simulink model "qr8x8"  (R2018b)
settings: Solver=VariableStepAuto  StartTime=0.0  StopTime=10.0  RelTol=1e-3
libraries: hdlsllib x71, simulink x16, dspmathops x1
(part 2 of 2)

== system qr8x8/QRdecomp/Q_col/Subsystem5/Subsystem5 ==
  i_bit : Inport
  j_bit : Inport  Port=2
  load : Inport  Port=3
  wr_en : Inport  Port=4
  Bit Concat : hdlsllib/Logic and Bit Operations/Bit Concat  numInputs=2
      settings: SourceProductName=HDL Coder  SourceProductBaseCode=HD
  Logical Operator : Logic  Operator=OR  AllPortsSameDT=off  OutDataTypeStr=boolean
  Logical Operator1 : Logic  Operator=OR  AllPortsSameDT=off  OutDataTypeStr=boolean
  Logical Operator2 : Logic  AllPortsSameDT=off  OutDataTypeStr=boolean
  din_sel : Outport
  en : Outport  Port=2
  wires:
  i_bit/1 -> Logical Operator/1, Bit Concat/2
  Logical Operator2/1 -> en/1
  wr_en/1 -> Logical Operator2/2
  Logical Operator1/1 -> Logical Operator2/1
  load/1 -> Logical Operator1/2
  Logical Operator/1 -> Logical Operator1/1
  Bit Concat/1 -> din_sel/1
  j_bit/1 -> Bit Concat/1, Logical Operator/2

== system qr8x8/QRdecomp/Q_col/Subsystem5/Subsystem6 ==
  i_bit : Inport
  j_bit : Inport  Port=2
  load : Inport  Port=3
  wr_en : Inport  Port=4
  Bit Concat : hdlsllib/Logic and Bit Operations/Bit Concat  numInputs=2
      settings: SourceProductName=HDL Coder  SourceProductBaseCode=HD
  Logical Operator : Logic  Operator=OR  AllPortsSameDT=off  OutDataTypeStr=boolean
  Logical Operator1 : Logic  Operator=OR  AllPortsSameDT=off  OutDataTypeStr=boolean
  Logical Operator2 : Logic  AllPortsSameDT=off  OutDataTypeStr=boolean
  din_sel : Outport
  en : Outport  Port=2
  wires:
  j_bit/1 -> Logical Operator/2, Bit Concat/1
  Bit Concat/1 -> din_sel/1
  Logical Operator/1 -> Logical Operator1/1
  load/1 -> Logical Operator1/2
  Logical Operator1/1 -> Logical Operator2/1
  wr_en/1 -> Logical Operator2/2
  Logical Operator2/1 -> en/1
  i_bit/1 -> Bit Concat/2, Logical Operator/1

== system qr8x8/QRdecomp/Q_col/Subsystem5/Subsystem7 ==
  i_bit : Inport
  j_bit : Inport  Port=2
  load : Inport  Port=3
  wr_en : Inport  Port=4
  Bit Concat : hdlsllib/Logic and Bit Operations/Bit Concat  numInputs=2
      settings: SourceProductName=HDL Coder  SourceProductBaseCode=HD
  Logical Operator : Logic  Operator=OR  AllPortsSameDT=off  OutDataTypeStr=boolean
  Logical Operator1 : Logic  Operator=OR  AllPortsSameDT=off  OutDataTypeStr=boolean
  Logical Operator2 : Logic  AllPortsSameDT=off  OutDataTypeStr=boolean
  din_sel : Outport
  en : Outport  Port=2
  wires:
  i_bit/1 -> Logical Operator/1, Bit Concat/2
  Logical Operator2/1 -> en/1
  wr_en/1 -> Logical Operator2/2
  Logical Operator1/1 -> Logical Operator2/1
  load/1 -> Logical Operator1/2
  Logical Operator/1 -> Logical Operator1/1
  Bit Concat/1 -> din_sel/1
  j_bit/1 -> Bit Concat/1, Logical Operator/2

== system qr8x8/QRdecomp/R_row/Subsystem/Subsystem ==
  sel : Inport
  load : Inport  Port=2
  din_i : Inport  Port=3
  "din_j " : Inport  Port=4
  din_load : Inport  Port=5
  Bit Slice : hdlsllib/Logic and Bit Operations/Bit Slice  lidx=1  ridx=1
  Bit Slice1 : hdlsllib/Logic and Bit Operations/Bit Slice  lidx=0  ridx=0
  Constant : Constant  Value=0  OutDataTypeStr=fixdt(1,32,25)  SampleTime=-1
  Logical Operator : Logic  Operator=XOR  AllPortsSameDT=off  OutDataTypeStr=boolean
  Switch : Switch  Criteria=u2 ~= 0
  Switch1 : Switch  Criteria=u2 ~= 0
  Switch2 : Switch  Criteria=u2 ~= 0
  din : Outport
  wires:
  Switch2/1 -> Switch1/3
  load/1 -> Switch1/2
  din_load/1 -> Switch1/1
  Switch1/1 -> din/1
  "din_j "/1 -> Switch/3
  Switch/1 -> Switch2/1
  Bit Slice/1 -> Logical Operator/1
  Bit Slice1/1 -> Logical Operator/2, Switch/2
  din_i/1 -> Switch/1
  sel/1 -> Bit Slice/1, Bit Slice1/1
  Logical Operator/1 -> Switch2/2
  Constant/1 -> Switch2/3

== system qr8x8/QRdecomp/R_row/Subsystem/Subsystem1 ==
  sel : Inport
  load : Inport  Port=2
  din_i : Inport  Port=3
  "din_j " : Inport  Port=4
  din_load : Inport  Port=5
  Bit Slice : hdlsllib/Logic and Bit Operations/Bit Slice  lidx=1  ridx=1
  Bit Slice1 : hdlsllib/Logic and Bit Operations/Bit Slice  lidx=0  ridx=0
  Constant : Constant  Value=0  OutDataTypeStr=fixdt(1,32,25)  SampleTime=-1
  Logical Operator : Logic  Operator=XOR  AllPortsSameDT=off  OutDataTypeStr=boolean
  Switch : Switch  Criteria=u2 ~= 0
  Switch1 : Switch  Criteria=u2 ~= 0
  Switch2 : Switch  Criteria=u2 ~= 0
  din : Outport
  wires:
  Constant/1 -> Switch2/3
  Logical Operator/1 -> Switch2/2
  sel/1 -> Bit Slice1/1, Bit Slice/1
  din_i/1 -> Switch/1
  Bit Slice1/1 -> Switch/2, Logical Operator/2
  Bit Slice/1 -> Logical Operator/1
  Switch/1 -> Switch2/1
  "din_j "/1 -> Switch/3
  Switch1/1 -> din/1
  din_load/1 -> Switch1/1
  load/1 -> Switch1/2
  Switch2/1 -> Switch1/3

== system qr8x8/QRdecomp/R_row/Subsystem/Subsystem2 ==
  sel : Inport
  load : Inport  Port=2
  din_i : Inport  Port=3
  "din_j " : Inport  Port=4
  din_load : Inport  Port=5
  Bit Slice : hdlsllib/Logic and Bit Operations/Bit Slice  lidx=1  ridx=1
  Bit Slice1 : hdlsllib/Logic and Bit Operations/Bit Slice  lidx=0  ridx=0
  Constant1 : Constant  Value=0  OutDataTypeStr=fixdt(1,32,25)  SampleTime=-1
  Logical Operator : Logic  Operator=XOR  AllPortsSameDT=off  OutDataTypeStr=boolean
  Switch : Switch  Criteria=u2 ~= 0
  Switch1 : Switch  Criteria=u2 ~= 0
  Switch2 : Switch  Criteria=u2 ~= 0
  din : Outport
  wires:
  Switch2/1 -> Switch1/3
  load/1 -> Switch1/2
  din_load/1 -> Switch1/1
  Switch1/1 -> din/1
  "din_j "/1 -> Switch/3
  Switch/1 -> Switch2/1
  Bit Slice/1 -> Logical Operator/1
  Bit Slice1/1 -> Logical Operator/2, Switch/2
  din_i/1 -> Switch/1
  sel/1 -> Bit Slice/1, Bit Slice1/1
  Logical Operator/1 -> Switch2/2
  Constant1/1 -> Switch2/3

== system qr8x8/QRdecomp/R_row/Subsystem/Subsystem3 ==
  sel : Inport
  load : Inport  Port=2
  din_i : Inport  Port=3
  "din_j " : Inport  Port=4
  din_load : Inport  Port=5
  Bit Slice : hdlsllib/Logic and Bit Operations/Bit Slice  lidx=1  ridx=1
  Bit Slice1 : hdlsllib/Logic and Bit Operations/Bit Slice  lidx=0  ridx=0
  Constant : Constant  Value=0  OutDataTypeStr=fixdt(1,32,25)  SampleTime=-1
  Logical Operator : Logic  Operator=XOR  AllPortsSameDT=off  OutDataTypeStr=boolean
  Switch : Switch  Criteria=u2 ~= 0
  Switch1 : Switch  Criteria=u2 ~= 0
  Switch2 : Switch  Criteria=u2 ~= 0
  din : Outport
  wires:
  Constant/1 -> Switch2/3
  Logical Operator/1 -> Switch2/2
  sel/1 -> Bit Slice1/1, Bit Slice/1
  din_i/1 -> Switch/1
  Bit Slice1/1 -> Switch/2, Logical Operator/2
  Bit Slice/1 -> Logical Operator/1
  Switch/1 -> Switch2/1
  "din_j "/1 -> Switch/3
  Switch1/1 -> din/1
  din_load/1 -> Switch1/1
  load/1 -> Switch1/2
  Switch2/1 -> Switch1/3

== system qr8x8/QRdecomp/R_row/Subsystem/Subsystem4 ==
  sel : Inport
  load : Inport  Port=2
  din_i : Inport  Port=3
  "din_j " : Inport  Port=4
  din_load : Inport  Port=5
  Bit Slice : hdlsllib/Logic and Bit Operations/Bit Slice  lidx=1  ridx=1
  Bit Slice1 : hdlsllib/Logic and Bit Operations/Bit Slice  lidx=0  ridx=0
  Constant : Constant  Value=0  OutDataTypeStr=fixdt(1,32,25)  SampleTime=-1
  Logical Operator : Logic  Operator=XOR  AllPortsSameDT=off  OutDataTypeStr=boolean
  Switch : Switch  Criteria=u2 ~= 0
  Switch1 : Switch  Criteria=u2 ~= 0
  Switch2 : Switch  Criteria=u2 ~= 0
  din : Outport
  wires:
  Switch2/1 -> Switch1/3
  load/1 -> Switch1/2
  din_load/1 -> Switch1/1
  Switch1/1 -> din/1
  "din_j "/1 -> Switch/3
  Switch/1 -> Switch2/1
  Bit Slice/1 -> Logical Operator/1
  Bit Slice1/1 -> Logical Operator/2, Switch/2
  din_i/1 -> Switch/1
  sel/1 -> Bit Slice/1, Bit Slice1/1
  Logical Operator/1 -> Switch2/2
  Constant/1 -> Switch2/3

== system qr8x8/QRdecomp/R_row/Subsystem/Subsystem5 ==
  sel : Inport
  load : Inport  Port=2
  din_i : Inport  Port=3
  "din_j " : Inport  Port=4
  din_load : Inport  Port=5
  Bit Slice : hdlsllib/Logic and Bit Operations/Bit Slice  lidx=1  ridx=1
  Bit Slice1 : hdlsllib/Logic and Bit Operations/Bit Slice  lidx=0  ridx=0
  Constant : Constant  Value=0  OutDataTypeStr=fixdt(1,32,25)  SampleTime=-1
  Logical Operator : Logic  Operator=XOR  AllPortsSameDT=off  OutDataTypeStr=boolean
  Switch : Switch  Criteria=u2 ~= 0
  Switch1 : Switch  Criteria=u2 ~= 0
  Switch2 : Switch  Criteria=u2 ~= 0
  din : Outport
  wires:
  Constant/1 -> Switch2/3
  Logical Operator/1 -> Switch2/2
  sel/1 -> Bit Slice1/1, Bit Slice/1
  din_i/1 -> Switch/1
  Bit Slice1/1 -> Switch/2, Logical Operator/2
  Bit Slice/1 -> Logical Operator/1
  Switch/1 -> Switch2/1
  "din_j "/1 -> Switch/3
  Switch1/1 -> din/1
  din_load/1 -> Switch1/1
  load/1 -> Switch1/2
  Switch2/1 -> Switch1/3

== system qr8x8/QRdecomp/R_row/Subsystem/Subsystem6 ==
  sel : Inport
  load : Inport  Port=2
  din_i : Inport  Port=3
  "din_j " : Inport  Port=4
  din_load : Inport  Port=5
  Bit Slice : hdlsllib/Logic and Bit Operations/Bit Slice  lidx=1  ridx=1
  Bit Slice1 : hdlsllib/Logic and Bit Operations/Bit Slice  lidx=0  ridx=0
  Constant : Constant  Value=0  OutDataTypeStr=fixdt(1,32,25)  SampleTime=-1
  Logical Operator : Logic  Operator=XOR  AllPortsSameDT=off  OutDataTypeStr=boolean
  Switch : Switch  Criteria=u2 ~= 0
  Switch1 : Switch  Criteria=u2 ~= 0
  Switch2 : Switch  Criteria=u2 ~= 0
  din : Outport
  wires:
  Switch2/1 -> Switch1/3
  load/1 -> Switch1/2
  din_load/1 -> Switch1/1
  Switch1/1 -> din/1
  "din_j "/1 -> Switch/3
  Switch/1 -> Switch2/1
  Bit Slice/1 -> Logical Operator/1
  Bit Slice1/1 -> Logical Operator/2, Switch/2
  din_i/1 -> Switch/1
  sel/1 -> Bit Slice/1, Bit Slice1/1
  Logical Operator/1 -> Switch2/2
  Constant/1 -> Switch2/3

== system qr8x8/QRdecomp/R_row/Subsystem/Subsystem7 ==
  sel : Inport
  load : Inport  Port=2
  din_i : Inport  Port=3
  "din_j " : Inport  Port=4
  din_load : Inport  Port=5
  Bit Slice : hdlsllib/Logic and Bit Operations/Bit Slice  lidx=1  ridx=1
  Bit Slice1 : hdlsllib/Logic and Bit Operations/Bit Slice  lidx=0  ridx=0
  Constant : Constant  Value=0  OutDataTypeStr=fixdt(1,32,25)  SampleTime=-1
  Logical Operator : Logic  Operator=XOR  AllPortsSameDT=off  OutDataTypeStr=boolean
  Switch : Switch  Criteria=u2 ~= 0
  Switch1 : Switch  Criteria=u2 ~= 0
  Switch2 : Switch  Criteria=u2 ~= 0
  din : Outport
  wires:
  Constant/1 -> Switch2/3
  Logical Operator/1 -> Switch2/2
  sel/1 -> Bit Slice1/1, Bit Slice/1
  din_i/1 -> Switch/1
  Bit Slice1/1 -> Switch/2, Logical Operator/2
  Bit Slice/1 -> Logical Operator/1
  Switch/1 -> Switch2/1
  "din_j "/1 -> Switch/3
  Switch1/1 -> din/1
  din_load/1 -> Switch1/1
  load/1 -> Switch1/2
  Switch2/1 -> Switch1/3

== system qr8x8/QRdecomp/R_row/Subsystem5/Subsystem ==
  i_bit : Inport
  j_bit : Inport  Port=2
  load : Inport  Port=3
  wr_en : Inport  Port=4
  Bit Concat : hdlsllib/Logic and Bit Operations/Bit Concat  numInputs=2
      settings: SourceProductName=HDL Coder  SourceProductBaseCode=HD
  Logical Operator : Logic  Operator=OR  AllPortsSameDT=off  OutDataTypeStr=boolean
  Logical Operator1 : Logic  Operator=OR  AllPortsSameDT=off  OutDataTypeStr=boolean
  Logical Operator2 : Logic  AllPortsSameDT=off  OutDataTypeStr=boolean
  din_sel : Outport
  en : Outport  Port=2
  wires:
  i_bit/1 -> Logical Operator/1, Bit Concat/2
  Logical Operator2/1 -> en/1
  wr_en/1 -> Logical Operator2/2
  Logical Operator1/1 -> Logical Operator2/1
  load/1 -> Logical Operator1/2
  Logical Operator/1 -> Logical Operator1/1
  Bit Concat/1 -> din_sel/1
  j_bit/1 -> Bit Concat/1, Logical Operator/2

== system qr8x8/QRdecomp/R_row/Subsystem5/Subsystem1 ==
  i_bit : Inport
  j_bit : Inport  Port=2
  load : Inport  Port=3
  wr_en : Inport  Port=4
  Bit Concat : hdlsllib/Logic and Bit Operations/Bit Concat  numInputs=2
      settings: SourceProductName=HDL Coder  SourceProductBaseCode=HD
  Logical Operator : Logic  Operator=OR  AllPortsSameDT=off  OutDataTypeStr=boolean
  Logical Operator1 : Logic  Operator=OR  AllPortsSameDT=off  OutDataTypeStr=boolean
  Logical Operator2 : Logic  AllPortsSameDT=off  OutDataTypeStr=boolean
  din_sel : Outport
  en : Outport  Port=2
  wires:
  j_bit/1 -> Logical Operator/2, Bit Concat/1
  Bit Concat/1 -> din_sel/1
  Logical Operator/1 -> Logical Operator1/1
  load/1 -> Logical Operator1/2
  Logical Operator1/1 -> Logical Operator2/1
  wr_en/1 -> Logical Operator2/2
  Logical Operator2/1 -> en/1
  i_bit/1 -> Bit Concat/2, Logical Operator/1

== system qr8x8/QRdecomp/R_row/Subsystem5/Subsystem2 ==
  i_bit : Inport
  j_bit : Inport  Port=2
  load : Inport  Port=3
  wr_en : Inport  Port=4
  Bit Concat : hdlsllib/Logic and Bit Operations/Bit Concat  numInputs=2
      settings: SourceProductName=HDL Coder  SourceProductBaseCode=HD
  Logical Operator : Logic  Operator=OR  AllPortsSameDT=off  OutDataTypeStr=boolean
  Logical Operator1 : Logic  Operator=OR  AllPortsSameDT=off  OutDataTypeStr=boolean
  Logical Operator2 : Logic  AllPortsSameDT=off  OutDataTypeStr=boolean
  din_sel : Outport
  en : Outport  Port=2
  wires:
  i_bit/1 -> Logical Operator/1, Bit Concat/2
  Logical Operator2/1 -> en/1
  wr_en/1 -> Logical Operator2/2
  Logical Operator1/1 -> Logical Operator2/1
  load/1 -> Logical Operator1/2
  Logical Operator/1 -> Logical Operator1/1
  Bit Concat/1 -> din_sel/1
  j_bit/1 -> Bit Concat/1, Logical Operator/2

== system qr8x8/QRdecomp/R_row/Subsystem5/Subsystem3 ==
  i_bit : Inport
  j_bit : Inport  Port=2
  load : Inport  Port=3
  wr_en : Inport  Port=4
  Bit Concat : hdlsllib/Logic and Bit Operations/Bit Concat  numInputs=2
      settings: SourceProductName=HDL Coder  SourceProductBaseCode=HD
  Logical Operator : Logic  Operator=OR  AllPortsSameDT=off  OutDataTypeStr=boolean
  Logical Operator1 : Logic  Operator=OR  AllPortsSameDT=off  OutDataTypeStr=boolean
  Logical Operator2 : Logic  AllPortsSameDT=off  OutDataTypeStr=boolean
  din_sel : Outport
  en : Outport  Port=2
  wires:
  j_bit/1 -> Logical Operator/2, Bit Concat/1
  Bit Concat/1 -> din_sel/1
  Logical Operator/1 -> Logical Operator1/1
  load/1 -> Logical Operator1/2
  Logical Operator1/1 -> Logical Operator2/1
  wr_en/1 -> Logical Operator2/2
  Logical Operator2/1 -> en/1
  i_bit/1 -> Bit Concat/2, Logical Operator/1

== system qr8x8/QRdecomp/R_row/Subsystem5/Subsystem4 ==
  i_bit : Inport
  j_bit : Inport  Port=2
  load : Inport  Port=3
  wr_en : Inport  Port=4
  Bit Concat : hdlsllib/Logic and Bit Operations/Bit Concat  numInputs=2
      settings: SourceProductName=HDL Coder  SourceProductBaseCode=HD
  Logical Operator : Logic  Operator=OR  AllPortsSameDT=off  OutDataTypeStr=boolean
  Logical Operator1 : Logic  Operator=OR  AllPortsSameDT=off  OutDataTypeStr=boolean
  Logical Operator2 : Logic  AllPortsSameDT=off  OutDataTypeStr=boolean
  din_sel : Outport
  en : Outport  Port=2
  wires:
  i_bit/1 -> Logical Operator/1, Bit Concat/2
  Logical Operator2/1 -> en/1
  wr_en/1 -> Logical Operator2/2
  Logical Operator1/1 -> Logical Operator2/1
  load/1 -> Logical Operator1/2
  Logical Operator/1 -> Logical Operator1/1
  Bit Concat/1 -> din_sel/1
  j_bit/1 -> Bit Concat/1, Logical Operator/2

== system qr8x8/QRdecomp/R_row/Subsystem5/Subsystem5 ==
  i_bit : Inport
  j_bit : Inport  Port=2
  load : Inport  Port=3
  wr_en : Inport  Port=4
  Bit Concat : hdlsllib/Logic and Bit Operations/Bit Concat  numInputs=2
      settings: SourceProductName=HDL Coder  SourceProductBaseCode=HD
  Logical Operator : Logic  Operator=OR  AllPortsSameDT=off  OutDataTypeStr=boolean
  Logical Operator1 : Logic  Operator=OR  AllPortsSameDT=off  OutDataTypeStr=boolean
  Logical Operator2 : Logic  AllPortsSameDT=off  OutDataTypeStr=boolean
  din_sel : Outport
  en : Outport  Port=2
  wires:
  j_bit/1 -> Logical Operator/2, Bit Concat/1
  Bit Concat/1 -> din_sel/1
  Logical Operator/1 -> Logical Operator1/1
  load/1 -> Logical Operator1/2
  Logical Operator1/1 -> Logical Operator2/1
  wr_en/1 -> Logical Operator2/2
  Logical Operator2/1 -> en/1
  i_bit/1 -> Bit Concat/2, Logical Operator/1

== system qr8x8/QRdecomp/R_row/Subsystem5/Subsystem6 ==
  i_bit : Inport
  j_bit : Inport  Port=2
  load : Inport  Port=3
  wr_en : Inport  Port=4
  Bit Concat : hdlsllib/Logic and Bit Operations/Bit Concat  numInputs=2
      settings: SourceProductName=HDL Coder  SourceProductBaseCode=HD
  Logical Operator : Logic  Operator=OR  AllPortsSameDT=off  OutDataTypeStr=boolean
  Logical Operator1 : Logic  Operator=OR  AllPortsSameDT=off  OutDataTypeStr=boolean
  Logical Operator2 : Logic  AllPortsSameDT=off  OutDataTypeStr=boolean
  din_sel : Outport
  en : Outport  Port=2
  wires:
  i_bit/1 -> Logical Operator/1, Bit Concat/2
  Logical Operator2/1 -> en/1
  wr_en/1 -> Logical Operator2/2
  Logical Operator1/1 -> Logical Operator2/1
  load/1 -> Logical Operator1/2
  Logical Operator/1 -> Logical Operator1/1
  Bit Concat/1 -> din_sel/1
  j_bit/1 -> Bit Concat/1, Logical Operator/2

== system qr8x8/QRdecomp/R_row/Subsystem5/Subsystem7 ==
  i_bit : Inport
  j_bit : Inport  Port=2
  load : Inport  Port=3
  wr_en : Inport  Port=4
  Bit Concat : hdlsllib/Logic and Bit Operations/Bit Concat  numInputs=2
      settings: SourceProductName=HDL Coder  SourceProductBaseCode=HD
  Logical Operator : Logic  Operator=OR  AllPortsSameDT=off  OutDataTypeStr=boolean
  Logical Operator1 : Logic  Operator=OR  AllPortsSameDT=off  OutDataTypeStr=boolean
  Logical Operator2 : Logic  AllPortsSameDT=off  OutDataTypeStr=boolean
  din_sel : Outport
  en : Outport  Port=2
  wires:
  j_bit/1 -> Logical Operator/2, Bit Concat/1
  Bit Concat/1 -> din_sel/1
  Logical Operator/1 -> Logical Operator1/1
  load/1 -> Logical Operator1/2
  Logical Operator1/1 -> Logical Operator2/1
  wr_en/1 -> Logical Operator2/2
  Logical Operator2/1 -> en/1
  i_bit/1 -> Bit Concat/2, Logical Operator/1

== matlab function qr8x8/QRdecomp/Q_col/i decoder ==
  data: bit0 output; bit1 output; bit2 output; bit3 output; bit4 output; bit5 output; bit6 output; i input; bit7 output
%#codegen
function [bit0,bit1,bit2,bit3,bit4,bit5,bit6,bit7] = fcn(i)

% switch to new state based on the value state register
switch (i)
    
    case 1
        bit7 = false;
        bit6 = false;
        bit5 = false;
        bit4 = false;
        bit3 = false;
        bit2 = false;
        bit1 = false;
        bit0 = true;
    case 2
        bit7 = false;
        bit6 = false;
        bit5 = false;
        bit4 = false;
        bit3 = false;
        bit2 = false;
        bit1 = true;
        bit0 = false;
    case 3
        bit7 = false;
        bit6 = false;
        bit5 = false;
        bit4 = false;
        bit3 = false;
        bit2 = true;
        bit1 = false;
        bit0 = false;
    case 4
        bit7 = false;
        bit6 = false;
        bit5 = false;
        bit4 = false;
        bit3 = true;
        bit2 = false;
        bit1 = false;
        bit0 = false;
    case 5
        bit7 = false;
        bit6 = false;
        bit5 = false;
        bit4 = true;
        bit3 = false;
        bit2 = false;
        bit1 = false;
        bit0 = false;
    case 6
        bit7 = false;
        bit6 = false;
        bit5 = true;
        bit4 = false;
        bit3 = false;
        bit2 = false;
        bit1 = false;
        bit0 = false;
    case 7
        bit7 = false;
        bit6 = true;
        bit5 = false;
        bit4 = false;
        bit3 = false;
        bit2 = false;
        bit1 = false;
        bit0 = false;
    case 8
        bit7 = true;
        bit6 = false;
        bit5 = false;
        bit4 = false;
        bit3 = false;
        bit2 = false;
        bit1 = false;
        bit0 = false;
        
    otherwise
        bit7 = false;
        bit6 = false;
        bit5 = false;
        bit4 = false;
        bit3 = false;
        bit2 = false;
        bit1 = false;
        bit0 = false;
end

== matlab function qr8x8/QRdecomp/Q_col/j decoder ==
  data: bit0 output; bit1 output; bit2 output; bit3 output; bit4 output; bit5 output; bit6 output; j input; bit7 output
%#codegen
function [bit0,bit1,bit2,bit3,bit4,bit5,bit6,bit7] = fcn(j)

% switch to new state based on the value state register
switch (j)
    case 0
        bit7 = false;
        bit6 = false;
        bit5 = false;
        bit4 = false;
        bit3 = false;
        bit2 = false;
        bit1 = false;
        bit0 = true;
    case 1
        bit7 = false;
        bit6 = false;
        bit5 = false;
        bit4 = false;
        bit3 = false;
        bit2 = false;
        bit1 = true;
        bit0 = false;
    case 2
        bit7 = false;
        bit6 = false;
        bit5 = false;
        bit4 = false;
        bit3 = false;
        bit2 = true;
        bit1 = false;
        bit0 = false;
    case 3
        bit7 = false;
        bit6 = false;
        bit5 = false;
        bit4 = false;
        bit3 = true;
        bit2 = false;
        bit1 = false;
        bit0 = false;
    case 4
        bit7 = false;
        bit6 = false;
        bit5 = false;
        bit4 = true;
        bit3 = false;
        bit2 = false;
        bit1 = false;
        bit0 = false;
    case 5
        bit7 = false;
        bit6 = false;
        bit5 = true;
        bit4 = false;
        bit3 = false;
        bit2 = false;
        bit1 = false;
        bit0 = false;
    case 6
        bit7 = false;
        bit6 = true;
        bit5 = false;
        bit4 = false;
        bit3 = false;
        bit2 = false;
        bit1 = false;
        bit0 = false;
    case 7
        bit7 = true;
        bit6 = false;
        bit5 = false;
        bit4 = false;
        bit3 = false;
        bit2 = false;
        bit1 = false;
        bit0 = false;
        
    otherwise
        bit7 = false;
        bit6 = false;
        bit5 = false;
        bit4 = false;
        bit3 = false;
        bit2 = false;
        bit1 = false;
        bit0 = false;
end

== matlab function qr8x8/QRdecomp/FSM ==
  data: svd_start input; ij_cnt_rst output; ij_cnt_trig output; UV_rd_sel output boolean; UV_wr_sel output; row_upd_srt output; UV_rd_lock output; qrd_done output; curr_state_DBG output; i input; j input; row_calc_done input; row_upd_done input
%#codegen
function [ij_cnt_rst, ij_cnt_trig, ...
    UV_rd_sel, UV_wr_sel, ...
    row_upd_srt, ...
    UV_rd_lock, ...
    qrd_done, ...
    curr_state_DBG] = ...
    fcn(svd_start, ...
    i, j, ...
    row_calc_done, row_upd_done)
% Moore State Machine

% y = f(x) : 
% all actions are state actions and 
% outputs are pure functions of state only 

% define states
S0_IDLE = ufi(0,5,0);
S1_READ_COL_J = ufi(1,5,0);
S2_READ_ROW = ufi(2,5,0);
S3_ROW_UPDATE = ufi(3,5,0);


% using persistent keyword to model state registers in hardware
persistent curr_state;
if isempty(curr_state)
    curr_state = S0_IDLE;   
end

% switch to new state based on the value state register
switch (curr_state)

    case S0_IDLE
        % decide next state value based on inputs
        ij_cnt_rst = false;
        ij_cnt_trig = false;
        UV_rd_sel = false;
        UV_wr_sel = false;
        row_upd_srt = false;
        qrd_done = false;
        UV_rd_lock = false;
        if (svd_start==true)
            ij_cnt_rst = true;
            UV_rd_lock = true;
            curr_state = S1_READ_COL_J;
        else
            curr_state = S0_IDLE;
        end

    case S1_READ_COL_J
        ij_cnt_rst = false;
        ij_cnt_trig = false;
        UV_rd_sel = true;
        UV_wr_sel = false;
        row_upd_srt = false;
        qrd_done = false;
        UV_rd_lock = true;
        curr_state = S2_READ_ROW;

    case S2_READ_ROW
        ij_cnt_rst = false;
        ij_cnt_trig = false;
        UV_rd_sel = false;
        UV_wr_sel = false;
        row_upd_srt = false;
        qrd_done = false;
        UV_rd_lock = true;
        if (row_calc_done)
            row_upd_srt = true;
            curr_state = S3_ROW_UPDATE;
        else
            curr_state = S2_READ_ROW;
        end

    case S3_ROW_UPDATE
        ij_cnt_rst = false;
        ij_cnt_trig = false;
        UV_rd_sel = false;
        row_upd_srt = false;
        UV_wr_sel = true;
        qrd_done = false;
        UV_rd_lock = true;
        if (row_upd_done)            
            if (i==7 && j==7)
                qrd_done = true;
                curr_state = S0_IDLE;
            else
                ij_cnt_trig = true;
                curr_state = S1_READ_COL_J;
            end
        else
            curr_state = S3_ROW_UPDATE;
        end

    otherwise
        ij_cnt_rst = false;
        ij_cnt_trig = false;
        UV_rd_sel = false;
        UV_wr_sel = false;
        row_upd_srt = false;
        qrd_done = false;
        UV_rd_lock = false;
        curr_state = S0_IDLE;
end

curr_state_DBG = curr_state;

== matlab function qr8x8/QRdecomp/R_row/i decoder ==
  data: bit0 output; bit1 output; bit2 output; bit3 output; bit4 output; bit5 output; bit6 output; i input; bit7 output
%#codegen
function [bit0,bit1,bit2,bit3,bit4,bit5,bit6,bit7] = fcn(i)

% switch to new state based on the value state register
switch (i)
    
    case 1
        bit7 = false;
        bit6 = false;
        bit5 = false;
        bit4 = false;
        bit3 = false;
        bit2 = false;
        bit1 = false;
        bit0 = true;
    case 2
        bit7 = false;
        bit6 = false;
        bit5 = false;
        bit4 = false;
        bit3 = false;
        bit2 = false;
        bit1 = true;
        bit0 = false;
    case 3
        bit7 = false;
        bit6 = false;
        bit5 = false;
        bit4 = false;
        bit3 = false;
        bit2 = true;
        bit1 = false;
        bit0 = false;
    case 4
        bit7 = false;
        bit6 = false;
        bit5 = false;
        bit4 = false;
        bit3 = true;
        bit2 = false;
        bit1 = false;
        bit0 = false;
    case 5
        bit7 = false;
        bit6 = false;
        bit5 = false;
        bit4 = true;
        bit3 = false;
        bit2 = false;
        bit1 = false;
        bit0 = false;
    case 6
        bit7 = false;
        bit6 = false;
        bit5 = true;
        bit4 = false;
        bit3 = false;
        bit2 = false;
        bit1 = false;
        bit0 = false;
    case 7
        bit7 = false;
        bit6 = true;
        bit5 = false;
        bit4 = false;
        bit3 = false;
        bit2 = false;
        bit1 = false;
        bit0 = false;
    case 8
        bit7 = true;
        bit6 = false;
        bit5 = false;
        bit4 = false;
        bit3 = false;
        bit2 = false;
        bit1 = false;
        bit0 = false;
        
    otherwise
        bit7 = false;
        bit6 = false;
        bit5 = false;
        bit4 = false;
        bit3 = false;
        bit2 = false;
        bit1 = false;
        bit0 = false;
end

== matlab function qr8x8/QRdecomp/R_row/j decoder ==
  data: bit0 output; bit1 output; bit2 output; bit3 output; bit4 output; bit5 output; bit6 output; j input; bit7 output
%#codegen
function [bit0,bit1,bit2,bit3,bit4,bit5,bit6,bit7] = fcn(j)

% switch to new state based on the value state register
switch (j)
    case 0
        bit7 = false;
        bit6 = false;
        bit5 = false;
        bit4 = false;
        bit3 = false;
        bit2 = false;
        bit1 = false;
        bit0 = true;
    case 1
        bit7 = false;
        bit6 = false;
        bit5 = false;
        bit4 = false;
        bit3 = false;
        bit2 = false;
        bit1 = true;
        bit0 = false;
    case 2
        bit7 = false;
        bit6 = false;
        bit5 = false;
        bit4 = false;
        bit3 = false;
        bit2 = true;
        bit1 = false;
        bit0 = false;
    case 3
        bit7 = false;
        bit6 = false;
        bit5 = false;
        bit4 = false;
        bit3 = true;
        bit2 = false;
        bit1 = false;
        bit0 = false;
    case 4
        bit7 = false;
        bit6 = false;
        bit5 = false;
        bit4 = true;
        bit3 = false;
        bit2 = false;
        bit1 = false;
        bit0 = false;
    case 5
        bit7 = false;
        bit6 = false;
        bit5 = true;
        bit4 = false;
        bit3 = false;
        bit2 = false;
        bit1 = false;
        bit0 = false;
    case 6
        bit7 = false;
        bit6 = true;
        bit5 = false;
        bit4 = false;
        bit3 = false;
        bit2 = false;
        bit1 = false;
        bit0 = false;
    case 7
        bit7 = true;
        bit6 = false;
        bit5 = false;
        bit4 = false;
        bit3 = false;
        bit2 = false;
        bit1 = false;
        bit0 = false;
        
    otherwise
        bit7 = false;
        bit6 = false;
        bit5 = false;
        bit4 = false;
        bit3 = false;
        bit2 = false;
        bit1 = false;
        bit0 = false;
end
